simulink model "generic_Truck_And_Trailer"  (R2025a)
settings: Solver=VariableStepAuto  StartTime=0.0  StopTime=350  FixedStep=0.01  MaxStep=0.001  RelTol=1e-3  EnableMultiTasking=on
libraries: TruckMaker4SL x250, simulink x1
(part 6 of 11)

== system generic_Truck_And_Trailer/TruckMaker/IPG Vehicle/CarAndTrailer/Forces/Suspension Forces/Stabi CreateBus CtrlOutOpt ==
  note: <Your model here>
  In : Inport
  Bus Creator{,1..3,11..14,19..22} (12 alike) : BusCreator  Inputs=4
  Bus Creator9 : BusCreator  Inputs=12
  Demux : Demux  Outputs=12
  Demux{2..5,10..13,18..21} (12 alike) : Demux
  Out : Outport
  wires:
  Demux/8 -> Demux13/1  "FR2"
  Demux19/1 -> Bus Creator20/1  "RR3 CtrlOutOpt0"
  Demux19/3 -> Bus Creator20/3  "RR3 CtrlOutOpt2"
  Demux18/4 -> Bus Creator19/4  "RL3 CtrlOutOpt3"
  Demux2/3 -> Bus Creator/3  "FL CtrlOutOpt2"
  Demux4/4 -> Bus Creator2/4  "RL CtrlOutOpt3"
  Demux3/2 -> Bus Creator1/2  "FR CtrlOutOpt1"
  Bus Creator11/1 -> Bus Creator9/5
  Demux2/4 -> Bus Creator/4  "FL CtrlOutOpt3"
  Demux/9 -> Demux18/1  "RL3"
  Demux10/3 -> Bus Creator11/3  "RL2 CtrlOutOpt2"
  Demux2/1 -> Bus Creator/1  "FL CtrlOutOpt0"
  Demux13/4 -> Bus Creator14/4  "FR2 CtrlOutOpt3"
  Demux19/4 -> Bus Creator20/4  "RR3 CtrlOutOpt3"
  Bus Creator1/1 -> Bus Creator9/2
  Bus Creator14/1 -> Bus Creator9/8
  Demux4/3 -> Bus Creator2/3  "RL CtrlOutOpt2"
  Demux2/2 -> Bus Creator/2  "FL CtrlOutOpt1"
  Demux5/1 -> Bus Creator3/1  "RR CtrlOutOpt0"
  Demux18/3 -> Bus Creator19/3  "RL3 CtrlOutOpt2"
  Demux12/1 -> Bus Creator13/1  "FL2 CtrlOutOpt0"
  Demux12/3 -> Bus Creator13/3  "FL2 CtrlOutOpt2"
  Bus Creator19/1 -> Bus Creator9/9
  Demux4/1 -> Bus Creator2/1  "RL CtrlOutOpt0"
  Demux10/1 -> Bus Creator11/1  "RL2 CtrlOutOpt0"
  Bus Creator/1 -> Bus Creator9/1
  Demux11/1 -> Bus Creator12/1  "RR2 CtrlOutOpt0"
  Demux20/1 -> Bus Creator21/1  "RL4 CtrlOutOpt0"
  Demux10/4 -> Bus Creator11/4  "RL2 CtrlOutOpt3"
  Bus Creator12/1 -> Bus Creator9/6
  Demux12/2 -> Bus Creator13/2  "FL2 CtrlOutOpt1"
  Demux11/3 -> Bus Creator12/3  "RR2 CtrlOutOpt2"
  Demux3/4 -> Bus Creator1/4  "FR CtrlOutOpt3"
  Demux18/2 -> Bus Creator19/2  "RL3 CtrlOutOpt1"
  Demux5/3 -> Bus Creator3/3  "RR CtrlOutOpt2"
  Demux19/2 -> Bus Creator20/2  "RR3 CtrlOutOpt1"
  Bus Creator20/1 -> Bus Creator9/10
  Demux20/2 -> Bus Creator21/2  "RL4 CtrlOutOpt1"
  Demux/7 -> Demux12/1  "FL2"
  Bus Creator2/1 -> Bus Creator9/3
  Demux/4 -> Demux5/1  "RR"
  Demux/1 -> Demux2/1  "FL"
  Demux20/4 -> Bus Creator21/4  "RL4 CtrlOutOpt3"
  Demux13/1 -> Bus Creator14/1  "FR2 CtrlOutOpt0"
  Demux/3 -> Demux4/1  "RL"
  Demux20/3 -> Bus Creator21/3  "RL4 CtrlOutOpt2"
  Demux3/1 -> Bus Creator1/1  "FR CtrlOutOpt0"
  Demux21/4 -> Bus Creator22/4  "RR4 CtrlOutOpt3"
  Demux11/4 -> Bus Creator12/4  "RR2 CtrlOutOpt3"
  Demux3/3 -> Bus Creator1/3  "FR CtrlOutOpt2"
  Demux18/1 -> Bus Creator19/1  "RL3 CtrlOutOpt0"
  Demux/10 -> Demux19/1  "RR3"
  Demux10/2 -> Bus Creator11/2  "RL2 CtrlOutOpt1"
  Demux12/4 -> Bus Creator13/4  "FL2 CtrlOutOpt3"
  Demux13/3 -> Bus Creator14/3  "FR2 CtrlOutOpt2"
  Demux4/2 -> Bus Creator2/2  "RL CtrlOutOpt1"
  Demux21/2 -> Bus Creator22/2  "RR4 CtrlOutOpt1"
  Demux5/2 -> Bus Creator3/2  "RR CtrlOutOpt1"
  Bus Creator3/1 -> Bus Creator9/4
  Demux21/3 -> Bus Creator22/3  "RR4 CtrlOutOpt2"
  Demux21/1 -> Bus Creator22/1  "RR4 CtrlOutOpt0"
  Demux/6 -> Demux11/1  "RR2"
  Demux/2 -> Demux3/1  "FR"
  Demux11/2 -> Bus Creator12/2  "RR2 CtrlOutOpt1"
  Demux13/2 -> Bus Creator14/2  "FR2 CtrlOutOpt1"
  Demux/5 -> Demux10/1  "RL2"
  Bus Creator13/1 -> Bus Creator9/7
  Demux5/4 -> Bus Creator3/4  "RR CtrlOutOpt3"
  In/1 -> Demux/1
  Bus Creator9/1 -> Out/1
  Demux/11 -> Demux20/1  "RL4"
  Bus Creator21/1 -> Bus Creator9/11
  Demux/12 -> Demux21/1  "RR4"
  Bus Creator22/1 -> Bus Creator9/12

== matlab function generic_Truck_And_Trailer/TruckMaker/Two_TRack_Model/EKF_ONE_TRACK ==
  data: z input; u input; xhat output; Q input; R input; Ts input; P output; Fyf output; Fyr output
function [xhat, P,Fyf,Fyr] = EKF_Bicycle_Full_NoBias(z, u, Q, R, Ts)
% EKF for One-Track / Bicycle Model (No IMU Bias)
% States: x = [vx; vy; r; Cf; Cr]
% Measurements: z = [ax; ay; vx; vy; r; wL; wR]

%% ---------------- Persistent safe initialization ----------------
persistent x Pk initialized

% Säker initialisering
if isempty(x)
    x = [15; 0; 0.05; 2e4; 2e4];  % vx, vy, r, Cf, Cr
end

if isempty(Pk)
    Pk = diag([1 1 0.05 4e4 4e4].^2); % 5x5
end

if isempty(initialized)
    initialized = true;
end


%% ---------------- Vehicle parameters ----------------


%% ---------------- Inputs ----------------
delta = u(1); % steering angle
Fx    = u(2)/Rw;    % longitudinal force

% PARAMETERS
m  = 6800;        %  mass
g  = 9.82;        % gravity contanst   
Jz = 12994.917;   % yaw interia
Rw = 0.49;          % wheel radius
width = 2.49;       % track width

p_cog  = [3.473; 0; 0.925];
p_fax  = [4.520; 0; 0.490];

p_rax  = [0.950; 0; 0.490];
p_imu  = [3.600; 0; 1.000];

lf = abs(p_fax(1)-p_cog(1));   % front CoG distance
lr = abs(p_cog(1)-p_rax(1));   % rear CoG distance
L  = lf + lr;
h  = p_cog(3);

Rfax = p_fax - p_imu; Rfax(3) = -p_imu(3);
Rrax = p_rax - p_imu; Rrax(3) = -p_imu(3);
Rcog = p_cog - p_imu;


% INPUTS
delta = u(1);                             % Average steering Angle (FL +FR)/2
T_rl  = u(2);                             % torque RL  
T_rr  = u(3);                             %torque RR
Rwheel = 0.49;                            % wheel radius
Fx_vehicle = (T_rl + T_rr)/Rwheel;        % longitudinal force

%% ---------------- States ----------------
vx = x(1); vy = x(2); r = x(3); Cf = x(4); Cr= x(5);

Rotf = [ cos(delta)     -sin(delta)     0;
         sin(delta)      cos(delta)     0;
             0              0           1];

v_cog = [vx; vy; 0];
omega = [0;0;r];

% Contact patch velocities
vf = Rotf.' * (v_cog + cross(omega,Rfax));
vr = v_cog + cross(omega,Rrax);

alpha_f = atan2(vf(2), max(abs(vf(1)),0.1));
alpha_r = atan2(vr(2), max(abs(vr(1)),0.1));

% Longitudinal accel estimate to compute the vertikel forces
dvx_temp = Fx_vehicle/m + vy*r;

% Normal forces
Ffz = m*g*lr/L - m*dvx_temp*h/L;
Frz = m*g*lf/L + m*dvx_temp*h/L;

% Tire forces
Fy_f = Cf * alpha_f * Ffz;
Fy_r = Cr * alpha_r * Frz;

% Full dynamics 
dvx = (Fx_vehicle - Fy_f*sin(delta))/m + vy*r;
dvy = (Fy_f*cos(delta) + Fy_r)/m - vx*r;
dr  = (lf*Fy_f*cos(delta) - lr*Fy_r)/Jz;

% State propagation
xdot = [dvx; dvy; dr; 0; 0];
x_pred = x + Ts*xdot;

%% ---------------- Jacobian F ----------------
F= zeros(5,5);
F(1,:) = [                                1 - (Cf*Ts*sin(delta)*(vy + lf*r))/(m*vx^2),              Ts*(r + (Cf*sin(delta))/(m*vx)),                   Ts*(vy + (Cf*lf*sin(delta))/(m*vx)),    -(Ts*sin(delta)*(delta - (vy + lf*r)/vx))/m,                            0];
F(2,:) = [  -Ts*(r - ((Cr*(vy - lr*r))/vx^2 + (Cf*cos(delta)*(vy + lf*r))/vx^2)/m),      1 - (Ts*(Cr/vx + (Cf*cos(delta))/vx))/m,    -Ts*(vx - ((Cr*lr)/vx - (Cf*lf*cos(delta))/vx)/m),     (Ts*cos(delta)*(delta - (vy + lf*r)/vx))/m,    -(Ts*(vy - lr*r))/(m*vx)];
F(3,:) = [-(Ts*((Cr*lr*(vy - lr*r))/vx^2 - (Cf*lf*cos(delta)*(vy + lf*r))/vx^2))/Jz, (Ts*((Cr*lr)/vx - (Cf*lf*cos(delta))/vx))/Jz, 1 - (Ts*((Cf*cos(delta)*lf^2)/vx + (Cr*lr^2)/vx))/Jz, (Ts*lf*cos(delta)*(delta - (vy + lf*r)/vx))/Jz, (Ts*lr*(vy - lr*r))/(Jz*vx)];
F(4,:) = [                                                                            0,                                              0,                                                      0,                                                 1,                            0];
F(5,:) = [                                                                            0,                                              0,                                                      0,                                                 0,                            1];


%% ---------------- Covariance prediction ----------------
P_pred = F*Pk*F' + Q;

%% ---------------- Measurement model ----------------
ax_hat = dvx -  vy*r;                % longitudinal accel
ay_hat = dvy + vx*r;                % lateral accel
vx_hat = vx;
vy_hat = vy;
r_hat  = r;
wL_hat = (vx - width/2 * r)/Rw;
wR_hat = (vx + width/2 * r)/Rw;

a_cog = [ax_hat; ay_hat; 0];
alpha_vec = [0;0;dr];

% Transform to IMU
a_imu = a_cog - cross(omega, cross(omega,Rcog))- cross(alpha_vec,Rcog);
v_imu = v_cog + cross(omega,Rcog);

z_hat = [a_imu(1:2);
         v_imu(1:2);
         alpha_vec(3);
         omega(3)];

%z_hat = [ax_hat; ay_hat; vx_hat; vy_hat; dr_hat r_hat; wL_hat; wR_hat];

%% ---------------- Measurement Jacobian H ----------------
H = zeros(size(z_hat,1),size(x,1));

%H = zeros(7,5);
H(1,:) = [                               1 - (Cf*Ts*sin(delta)*(vy + lf*r))/(m*vx^2),         Ts*(r + (Cf*sin(delta))/(m*vx)) - r,                      Ts*(vy + (Cf*lf*sin(delta))/(m*vx)) - vy, -(Ts*sin(delta)*(delta - (vy + lf*r)/vx))/m,                            0];
H(2,:) = [-Ts*(r - ((Cr*(vy - lr*r))/vx^2 + (Cf*cos(delta)*(vy + lf*r))/vx^2)/m), 1 - (Ts*(Cr/vx_eff + (Cf*cos(delta))/vx))/m, vx - Ts*(vx - ((Cr*lr)/vx - (Cf*lf*cos(delta))/vx)/m),  (Ts*cos(delta)*(delta - (vy + lf*r)/vx))/m, -(Ts*(vy - lr*r))/(m*vx)];
H(3,:) = [                                                                             1,                                               0,                                                                 0,                                               0,            0];
H(4,:) = [                                                                             0,                                               1,                                                                 0,                                               0,            0];
H(5,:) = [                                                                             0,                                               0,                                                                 0,                                               0,            0];
H(6,:) = [                                                                             0,                                               0,                                                                 1,                                               0,            0];
H(7,:) = [                                                                             1/Rw,                                            0,                                                     -width/(2*Rw),                                               0,            0];
H(8,:) = [                                                                             1/Rw,                                            0,                                                      width/(2*Rw),                                               0,            0];

%% ---------------- EKF update ----------------
S = H*P_pred*H' + R;
K = P_pred*H'/S;

x = x_pred + K*(z - z_hat);
Pk = P_pred - K*S*K';

%% ---------------- Output ----------------
xhat = x;
P = Pk;

end

== matlab function generic_Truck_And_Trailer/TruckMaker/Two_TRack_Model/MATLAB Function2 ==
  data: z input; u input; vx output; Ts input; vy output; wz output; Cf_est output; Cr_est output; Fyf output; Fyr output
function [vx, vy, wz, Cf_est, Cr_est, Fyf, Fyr] = AdaptiveOneTrackCFCR(z, u, Ts)
% Adaptive one-track model for online estimation of front/rear cornering stiffness
%
% Inputs:
%   z  = [ax; ay; vx; vy; wz] -> sensor measurements
%   u  = [delta; Fx]          -> steering angle (rad), longitudinal force (N)
%   Ts -> sampling time (s)
%
% Outputs:
%   vx, vy, wz      -> vehicle states (m/s, m/s, rad/s)
%   Cf_est, Cr_est  -> estimated front/rear cornering stiffness (N/rad)
%   Fyf, Fyr        -> lateral forces (N)

persistent Cf Cr vx_prev vy_prev wz_prev

%% ---------------- Initialization ----------------
if isempty(vx_prev)
    vx_prev = z(3); vy_prev = z(4); wz_prev = z(5);
end
if isempty(Cf)
    Cf = 15000;  % initial guess
    Cr = 15000;
end

%% ---------------- Vehicle parameters ----------------
m  = 7000;      % mass [kg]
Jz = 14232.357; % yaw inertia [kg*m^2]
lf = 1.12;      % front CoG to axle [m]
lr = 2.45;      % rear CoG to axle [m]
Rw = 0.49;      % wheel radius [m]
track = 2.49;   % track width [m]

%% ---------------- Inputs ----------------
delta = u(1); % steering [rad]
Fx    = u(2); % longitudinal force [N]

%% ---------------- States from sensors ----------------
vx = z(3); 
vy = z(4); 
wz = z(5);

% Protect low velocity
vx_eff = max(abs(vx), 1);

%% ---------------- Slip angles ----------------
alpha_f = (vy + lf*wz)/vx_eff - delta;
alpha_r = (vy - lr*wz)/vx_eff;

%% ---------------- Lateral forces ----------------
Fyf = -Cf * alpha_f;
Fyr = -Cr * alpha_r;

%% ---------------- Approximate derivatives ----------------
% simple backward difference
dv_y = (vy - vy_prev)/Ts;
dw_z = (wz - wz_prev)/Ts;

%% ---------------- Regression for Cf/Cr ----------------
% Linear regression: y = Phi * [Cf; Cr]
y   = [m*(dv_y + vx*wz); Jz*dw_z];
Phi = [alpha_f, alpha_r; lf*alpha_f, -lr*alpha_r];

% Adaptive gain
gamma = 1e3;

theta = [Cf; Cr] + gamma * Phi' * (y - Phi*[Cf; Cr]) * Ts;

% Limit to physical range
Cf = theta(1);%max(min(theta(1), 1e5), 5000);
Cr = theta(2);%max(min(theta(2), 1e5), 5000);

Cf_est = Cf;
Cr_est = Cr;

%% ---------------- Recompute lateral forces ----------------
Fyf = Cf_est * alpha_f;
Fyr = -Cr_est * alpha_r;

%% ---------------- Update previous states ----------------
vx_prev = vx;
vy_prev = vy;
wz_prev = wz;

end

== matlab function generic_Truck_And_Trailer/TruckMaker/Comparison Block Forces /Comparison Functions  ==
  data: Vec_v input; alpha_f output; Car_w input; delta_f input; Toe_angle input; alpha_r output; CyF input; CyR input; Fy output; Vx_wheel output; Vy_wheel output
function [alpha_f, alpha_r, Fy, Vx_wheel, Vy_wheel] = tire_model_4W_vehicleFrame(Vec_v, Car_w, delta_f,Toe_angle, CyF, CyR)
%TIRE_MODEL_4W_VEHICLEFRAME
%  Beräknar slipvinklar och lateral forces för ett 4-hjuls fordon
%  
%  Input:
%    Vec_v   - [3x1] Vehicle velocity i vehicle frame [Vx; Vy; Vz]
%    Car_w   - [3x1] Vehicle angular rates i vehicle frame [rollRate; pitchRate; yawRate]
%    delta_f - [2x1] Framhjul styrvinklar [delta_FL; delta_FR] (rad)
%    CyF     - [2x1] Framhjul cornering stiffness per wheel
%    CyR     - [2x1] Bakhjul cornering stiffness per wheel
%
%  Output:
%    alpha_f - [2x1] Slipvinkel framhjul [rad]
%    alpha_r - [2x1] Slipvinkel bakhjul [rad]
%    Fy      - [4x1] Lateral force per wheel [N]
%    Vx_wheel, Vy_wheel - [4x1] Hjulhastigheter i hjulens frame

%% ================= PARAMETERS =================
eps_v  = 0.1;   % min velocity för slipvinkel
g = 9.82;       % gravitation [m/s^2]
load_front_axle = 4805.882;   
load_rear_axle  = 2194.118;   

%% ================= GEOMETRY =================
% Kontaktpunkter i vehicle frame
tire_contact_point_FL = [4.52;  1.05; 0]; 
tire_contact_point_FR = [4.52; -1.05; 0];
tire_contact_point_RL = [0.95;  1.05; 0];
tire_contact_point_RR = [0.95; -1.05; 0];

% Reference point (IMU/vehicle CoM)
Vec_coor = [3.6; 0; 1];

% Vektorer från CoM till hjul
rFL = tire_contact_point_FL - Vec_coor;
rFR = tire_contact_point_FR - Vec_coor;
rRL = tire_contact_point_RL - Vec_coor;
rRR = tire_contact_point_RR - Vec_coor;

%% ================= CONTACT PATCH VELOCITY =================
V_FL = Vec_v + cross(Car_w, rFL);
V_FR = Vec_v + cross(Car_w, rFR);
V_RL = Vec_v + cross(Car_w, rRL);
V_RR = Vec_v + cross(Car_w, rRR);

%% ================= TRANSFORM TO WHEEL FRAME =================
% 2D rotation för framhjul
R_FL = [cos(delta_f(1)), sin(delta_f(1));
       -sin(delta_f(1)), cos(delta_f(1))];

R_FR = [cos(delta_f(2)), sin(delta_f(2));
       -sin(delta_f(2)), cos(delta_f(2))];

% Bakhjul (delta=0)
R_RL = eye(2);
R_RR = eye(2);

% Transformera
V_FL_local = R_FL * V_FL(1:2);
V_FR_local = R_FR * V_FR(1:2);
V_RL_local = R_RL * V_RL(1:2);
V_RR_local = R_RR * V_RR(1:2);


Vx_wheel = [V_FL_local(1); V_FR_local(1); V_RL_local(1); V_RR_local(1)];
Vy_wheel = [V_FL_local(2); V_FR_local(2); V_RL_local(2); V_RR_local(2)];

%% ================= SLIP ANGLES =================
Vx_safe = max(abs(Vx_wheel), eps_v);  % förhindrar division med 0
alpha = atan2(Vy_wheel, Vx_safe);

% Fram och bak separering
alpha_f = alpha(1:2); % - Toe_angle(1:2);
alpha_r = alpha(3:4);% + Toe_angle(3:4).*[1;-1];

%% ================= CORNERING STIFFNESS =================
Cy_FL = CyF(1) * load_front_axle * g / 2;
Cy_FR = CyF(2) * load_front_axle * g / 2;

Cy_RL = CyR(1) * load_rear_axle  * g / 2;
Cy_RR = CyR(2) * load_rear_axle  * g / 2;

Cy = [Cy_FL; Cy_FR; Cy_RL; Cy_RR];

%% ================= LATERAL FORCES =================
Fy = -Cy .* alpha;

end

== matlab function generic_Truck_And_Trailer/TruckMaker/Two_TRack_Model/MATLAB Function3 ==
  data: z input; u input; xhat output; Q input; R input; Ts input; P output; sensor_pos input; F_wheel_pos input; R_wheel_pos input
function [xhat,P] = UKF_5state_4W(z,u,Q,R,Ts,sensor_pos,F_wheel_pos,R_wheel_pos)
% UKF for 4-wheel vehicle
% States: x = [vx; vy; wz; CyF; CyR]
% Measurements: z = [ax; ay; vx; vy; wz; wFL; wFR; wRL; wRR]

persistent x Pk
if isempty(x)
    x = [15; 0; 0.05; 4e4; 4e4]; % initial state
end
if isempty(Pk)
    Pk = diag([1 1 0.01 1e6 1e6]);
end

%% Vehicle parameters
m  = 7000;
Jz = 14232.357;
Rw = 0.49;
g  = 9.82;
track = 2.49;

n = length(x); % state dimension

delta = u(1);      % steering input
Fx_in = u(2)/Rw;   % longitudinal force / wheel radius

%% UKF weights (old style)
W0 = 1 - n/3;
Wi = (1-W0)/(2*n);
gamma = sqrt(n/(1-W0));

%% Sigma points
S = chol(Pk,'lower');
X = zeros(n,2*n+1);
X(:,1) = x;
for i=1:n
    X(:,i+1)   = x + gamma*S(:,i);
    X(:,i+1+n) = x - gamma*S(:,i);
end

%% ------------------- PREDICTION -------------------
X_pred = zeros(n,2*n+1);

for k=1:2*n+1
    vx  = X(1,k);
    vy  = X(2,k);
    wz  = X(3,k);
    CyF = X(4,k);
    CyR = X(5,k);

    Car_v = [vx; vy; 0];
    Car_w = [wx; wy; wz];

    % ---- Wheel velocities at contact patch ----
    V_FL = Car_v + cross(Car_w, F_wheel_pos.FL);
    V_FR = Car_v + cross(Car_w, F_wheel_pos.FR);
    V_RL = Car_v + cross(Car_w, R_wheel_pos.RL);
    V_RR = Car_v + cross(Car_w, R_wheel_pos.RR);

    % ---- Rotate front wheels to wheel frame ----
    R_FL = [ cos(delta)  sin(delta) 0;
            -sin(delta)  cos(delta) 0;
             0           0          1];
    R_FR = R_FL;

    VwfL = R_FL * V_FL;
    VwfR = R_FR * V_FR;

    VwrL = V_RL; % rear wheels no steering
    VwrR = V_RR;

    % ---- Slip angles ----
    alpha_FL = atan2(VwfL(2), VwfL(1));
    alpha_FR = atan2(VwfR(2), VwfR(1));
    alpha_RL = atan2(VwrL(2), VwrL(1));
    alpha_RR = atan2(VwrR(2), VwrR(1));

    % ---- Lateral forces ----
    Fy_FL = -CyF * alpha_FL;
    Fy_FR = -CyF * alpha_FR;
    Fy_RL = -CyR * alpha_RL;
    Fy_RR = -CyR * alpha_RR;

    % Total lateral force & yaw moment
    Fy_total = Fy_FL + Fy_FR + Fy_RL + Fy_RR;
    Mz = F_wheel_pos.FL(1)*Fy_FL + F_wheel_pos.FR(1)*Fy_FR + ...
         R_wheel_pos.RL(1)*Fy_RL + R_wheel_pos.RR(1)*Fy_RR;

    % ---- Dynamics ----
    dvx = Fx_in/m + vy*wz;
    dvy = Fy_total/m - vx*wz;
    dwz = Mz / Jz;

    % Propagate state
    X_pred(:,k) = [vx + Ts*dvx;
                   vy + Ts*dvy;
                   wz + Ts*dwz;
                   CyF;
                   CyR];
end

%% Predicted mean
x_pred = W0*X_pred(:,1);
for k=2:2*n+1
    x_pred = x_pred + Wi*X_pred(:,k);
end

%% Predicted covariance
P_pred = Q;
for k=1:2*n+1
    w = Wi; if k==1, w=W0; end
    dx = X_pred(:,k) - x_pred;
    P_pred = P_pred + w*(dx*dx');
end

%% ------------------- MEASUREMENT -------------------
m_dim = length(z);
Z = zeros(m_dim,2*n+1);

for k=1:2*n+1
    vx  = X_pred(1,k);
    vy  = X_pred(2,k);
    wz  = X_pred(3,k);
    CyF = X_pred(4,k);
    CyR = X_pred(5,k);

    Car_v = [vx; vy; 0];
    Car_w = [0; 0; wz];

    % Velocity at sensor
    V_sensor = Car_v + cross(Car_w, sensor_pos);

    % Acceleration at sensor (approx)
    ax_s = Fx_in/m + vy*wz;
    ay_s = ( -CyF*(atan2(Car_v(2)+wz*F_wheel_pos.FL(2),Car_v(1))) ...
           -CyF*(atan2(Car_v(2)+wz*F_wheel_pos.FR(2),Car_v(1))) ...
           -CyR*(atan2(Car_v(2)+wz*R_wheel_pos.RL(2),Car_v(1))) ...
           -CyR*(atan2(Car_v(2)+wz*R_wheel_pos.RR(2),Car_v(1))) )/m;
    az_s = 0;

    % Wheel speeds
    wFL = V_FL(1)/Rw;
    wFR = V_FR(1)/Rw;
    wRL = V_RL(1)/Rw;
    wRR = V_RR(1)/Rw;

    Z(:,k) = [ax_s; ay_s; vx; vy; wz; wFL; wFR; wRL; wRR];
end

% Predicted measurement mean
z_pred = W0*Z(:,1);
for k=2:2*n+1
    z_pred = z_pred + Wi*Z(:,k);
end

% Measurement covariance & cross-covariance
S_cov = R;
Pxz   = zeros(n,m_dim);
for k=1:2*n+1
    w = Wi; if k==1, w=W0; end
    dz = Z(:,k) - z_pred;
    dx = X_pred(:,k) - x_pred;
    S_cov = S_cov + w*(dz*dz');
    Pxz   = Pxz + w*(dx*dz');
end

% Kalman gain
K = Pxz / (S_cov + 1e-6*eye(m_dim));

% Update
x  = x_pred + K*(z - z_pred);
Pk = P_pred - K*S_cov*K';

xhat = x;
P    = Pk;

end



%%%%%%%%%%%%%%%%%%%%%%%
function [alpha_f, alpha_r, Ffy, Fry, ...
          VfL, VfR, VrL, VrR] = tire_model_4W( ...
          Car_v, Car_w, delta_f, CyF, CyR)

% ------------------------------------------------------------
% INPUTS
% Car_v   = [vx; vy; vz]      (vehicle body frame)
% Car_w   = [0; 0; wz]        (vehicle body frame)
% delta_f = [delta_L; delta_R] (front steering angles)
% CyF     = [Cy_FL; Cy_FR]
% CyR     = [Cy_RL; Cy_RR]
%
% OUTPUTS
% alpha_f = [alpha_FL; alpha_FR]
% alpha_r = [alpha_RL; alpha_RR]
% Ffy     = [Fy_FL; Fy_FR]
% Fry     = [Fy_RL; Fy_RR]
% VwfL etc = velocities in wheel frame
% ------------------------------------------------------------

%% ================= PARAMETERS =================
R = 0.49;                 % wheel radius
g = 9.82;

load_front_axle = 4805.882;
load_rear_axle  = 2194.118;

%% ================= GEOMETRY =================
% Wheel centers in vehicle body frame
tire_coor_Fl = [4.52;  1.05; 0.49];
tire_coor_FR = [4.52; -1.05; 0.49];
tire_coor_Rl = [0.95;  1.05; 0.49];
tire_coor_RR = [0.95; -1.05; 0.49];

Car_coor = [3.6; 0; 1];

% Position vectors CG → wheel center
rFl = tire_coor_Fl - Car_coor;
rFR = tire_coor_FR - Car_coor;
rRl = tire_coor_Rl - Car_coor;
rRR = tire_coor_RR - Car_coor;

% Move to CONTACT PATCH
rFl = rFl + [0;0;-R];
rFR = rFR + [0;0;-R];
rRl = rRl + [0;0;-R];
rRR = rRR + [0;0;-R];

%% ================= VELOCITIES AT CONTACT =================
VfL = Car_v + cross(Car_w, rFl);
VfR = Car_v + cross(Car_w, rFR);
VrL = Car_v + cross(Car_w, rRl);
VrR = Car_v + cross(Car_w, rRR);

%% ================= ROTATE TO WHEEL FRAME =================
% Front left
R_FL = [ cos(delta_f(1))  -sin(delta_f(1)) 0;
        sin(delta_f(1))  cos(delta_f(1)) 0;
         0                0               1];

% Front right
R_FR = [ cos(delta_f(2))  -sin(delta_f(2)) 0;
       sin(delta_f(2))  cos(delta_f(2)) 0;
         0                0               1];

VfL = R_FL * VfL;
VfR = R_FR * VfR;

% Rear wheels (no steering)
%VrL = VrL;
%VrR = VrR;

%% ================= SLIP ANGLES =================
alpha_FL = atan2(VfL(2), VfL(1)); %- delta_f(1);
alpha_FR = atan2(VfR(2), VfR(1));%- delta_f(2);

alpha_RL = atan2(VrL(2), VrL(1));
alpha_RR = atan2(VrR(2), VrR(1));

alpha_f = [alpha_FL; alpha_FR];
alpha_r = [alpha_RL; alpha_RR];

%% ================= CORNERING STIFFNESS =================
Cy_FL = CyF(1) * load_front_axle * g / 2;
Cy_FR = CyF(2) * load_front_axle * g / 2;

Cy_RL = CyR(1) * load_rear_axle * g/2;
Cy_RR = CyR(2) * load_rear_axle * g/2;

%% ================= LATERAL FORCES =================
Fy_FL = -Cy_FL * alpha_FL;
Fy_FR = -Cy_FR * alpha_FR;

Fy_RL = -Cy_RL * alpha_RL;
Fy_RR = -Cy_RR * alpha_RR;

Ffy = [Fy_FL; Fy_FR];
Fry = [Fy_RL; Fy_RR];

end

== matlab function generic_Truck_And_Trailer/TruckMaker/MATLAB Function1 ==
  data: CarVelocity input; CarOmega input; V_FL output; WheelCamberAngle input
function V_FL = fcn(CarVelocity, CarOmega, WheelCamberAngle)

== matlab function generic_Truck_And_Trailer/TruckMaker/Two_TRack_Model/Two Track Model ==
  data: z input; u input; Q input; R input; xhat output; Ts input; P_out output; Fy_mean output; alpha_mean output; V_FL_whl output; V_FR_whl output; V_RL_whl output; V_RR_whl output
function [xhat,P_out,Fy_mean,alpha_mean,...
          V_FL_whl,V_FR_whl,V_RL_whl,V_RR_whl] ...
          = UKF_4Wheel(z,u,Q,R,Ts)

persistent x P

%% ================= INIT =================
if isempty(x)
    x = [15; 0; 0.01; 4; 4; 4; 4];
end

if isempty(P)
    P = diag([1 1 0.01 1e4 1e4 1e4 1e4]);
end

n = length(x);
m = length(z);

%% ================= VEHICLE =================
m_car = 7000;
Jz = 14232.357;
lf = 4.52;
lr = 0.95;
R_w = 0.49;
track=2.10;

%% ================= INPUTS =================
delta_FL = u(1);
delta_FR = u(2);
delta_RL = 0;
delta_RR = 0;

Fx_FL = u(5)/R_w;
Fx_FR = u(6)/R_w;
Fx_RL = u(7)/R_w;
Fx_RR = u(8)/R_w;

%% ================= ROTATION MATRICES =================
R_FL = [cos(delta_FL) sin(delta_FL);
       -sin(delta_FL) cos(delta_FL)];

R_FR = [cos(delta_FR) sin(delta_FR);
       -sin(delta_FR) cos(delta_FR)];

R_RL = eye(2);
R_RR = eye(2);

%% ================= GEOMETRY =================
tire_FL = [lf;  1.05; 0];
tire_FR = [lf; -1.05; 0];
tire_RL = [lr;  1.05; 0];
tire_RR = [lr; -1.05; 0];

CoM = [3.6; 0; 1];  % Ändra koor till COM (Jobba i CoG)  

rFL = tire_FL - CoM;
rFR = tire_FR - CoM;
rRL = tire_RL - CoM;
rRR = tire_RR - CoM;

%% ================= UKF =================
W0 = 1 - n/3;
Wi = (1 - W0)/(2*n);
gamma = sqrt(n/(1-W0));

%P = (P+P')/2 + 1e-9*eye(n); 
S = chol(P,'lower'); %% kolla upp den igen 

X = zeros(n,2*n+1);
X(:,1) = x;

for i=1:n
    X(:,i+1)   = x + gamma*S(:,i);
    X(:,i+1+n) = x - gamma*S(:,i);
end

%% ================= PROPAGATION =================
X_pred = zeros(n,2*n+1);
Fy_sigma = zeros(4,2*n+1);
alpha_sigma = zeros(4,2*n+1);
% R; M; Jz
for k=1:2*n+1

    vx = X(1,k);
    vy = X(2,k);
    r  = X(3,k);

    Cf_FL = X(4,k);
    Cf_FR = X(5,k);
    Cr_RL = X(6,k);
    Cr_RR = X(7,k);

    % ===== FIX 1: korrekt vx_safe =====
    %vx_safe = vx;

    Vc = [vx; vy; 0]; % vehilce Frame 
    omega = [0;0;r];

    V_FL = Vc + cross(omega,rFL);
    V_FR = Vc + cross(omega,rFR);
    V_RL = Vc + cross(omega,rRL);
    V_RR = Vc + cross(omega,rRR);

    V_FL_l = R_FL*V_FL(1:2);
    V_FR_l = R_FR*V_FR(1:2);
    V_RL_l = V_RL(1:2);
    V_RR_l = V_RR(1:2);
    
    %============Side Slip Vinkel på respektiv däck ==================
    alpha_FL = atan2(V_FL_l(2),max(abs(V_FL_l(1)),0.1));
    alpha_FR = atan2(V_FR_l(2),max(abs(V_FR_l(1)),0.1));
    alpha_RL = atan2(V_RL_l(2),max(abs(V_RL_l(1)),0.1));
    alpha_RR = atan2(V_RR_l(2),max(abs(V_RR_l(1)),0.1));


    %===================Forces==============================
    Fy_FL = -Cf_FL*alpha_FL;
    Fy_FR = -Cf_FR*alpha_FR;
    Fy_RL = -Cr_RL*alpha_RL;
    Fy_RR = -Cr_RR*alpha_RR;


    % Transformerta dessa krafter till kroppens FRAME
    F_FL = R_FL'*[Fx_FL;Fy_FL];
    F_FR = R_FR'*[Fx_FR;Fy_FR];
    F_RL = [Fx_RL;Fy_RL];
    F_RR = [Fx_RR;Fy_RR];

    Fx_sum = F_FL(1)+F_FR(1)+F_RL(1)+F_RR(1);
    Fy_sum = F_FL(2)+F_FR(2)+F_RL(2)+F_RR(2);

    dvx = Fx_sum/m_car + vy*r; % andra terma roteradnde koordinat system 
    dvy = Fy_sum/m_car - vx*r; 

%dW = truck.Jinv * (cross(R1, RotW1*F1) + cross(R2, RotW2*F2) 
                    % + cross(R3, F3) + cross(R4, F4));

    % ===== FIX 2: korrekt  eller ej fråga Axel  yaw moment =====
    % !!!!!!!!!!
    Mz = (lf-CoM(1))*(F_FL(2)+F_FR(2)) - (CoM(1)-lr)*(F_RL(2)+F_RR(2)) ... 
        + (track/2)*(F_FR(1)-F_FL(1)) + (track/2)*(F_RR(1)-F_RL(1));
    dr = Mz / Jz;

    X_pred(:,k) = [vx+dvx*Ts;
                   vy+dvy*Ts;
                   r+dr*Ts;
                   Cf_FL;
                   Cf_FR;
                   Cr_RL;
                   Cr_RR];

    Fy_sigma(:,k)    = [F_FL(2);F_FR(2);F_RL(2);F_RR(2)];
    alpha_sigma(:,k) = [alpha_FL;alpha_FR;alpha_RL;alpha_RR];
end

W = [W0 repmat(Wi,1,2*n)];
%x_pred = X_pred*W';
Fy_mean = Fy_sigma*W';
alpha_mean = alpha_sigma*W';
%% Predicted mean
x_pred = W0*X_pred(:,1);
for k=2:2*n+1
    x_pred = x_pred + Wi*X_pred(:,k);
end

%% ================= COVARIANCE =================
% P_pred = Q*Ts;
% for k=1:2*n+1
%     dx = X_pred(:,k)-x_pred;
%     P_pred = P_pred + W(k)*(dx*dx');
% end

%% Predicted covariance
P_pred = Q*Ts;
for k=1:2*n+1
    w = (k==1)*W0 + (k>1)*Wi;
    dx = X_pred(:,k) - x_pred;
    P_pred = P_pred + w*(dx*dx');
end
%% ================= MEASUREMENT =================
Z_sigma = zeros(m,2*n+1);

for k=1:2*n+1

    vx = X_pred(1,k);
    vy = X_pred(2,k);
    r  = X_pred(3,k);

    %Cf_FL = X_pred(4,k);
    %Cf_FR = X_pred(5,k);
    %Cr_RL = X_pred(6,k);
    %Cr_RR = X_pred(7,k);


    vx_safe = abs(vx);

    Vc = [vx_safe;vy;0];
    omega = [0;0;r];

    V_FL = Vc + cross(omega,rFL);
    V_FR = Vc + cross(omega,rFR);
    V_RL = Vc + cross(omega,rRL);
    V_RR = Vc + cross(omega,rRR);

    V_FL_l = R_FL*V_FL(1:2);
    V_FR_l = R_FR*V_FR(1:2);
    V_RL_l = V_RL(1:2);
    V_RR_l = V_RR(1:2);

     %============Side Slip Vinkel på respektiv däck ==================
    alpha_FL = atan2(V_FL_l(2),max(abs(V_FL_l(1)),0.1));
    alpha_FR = atan2(V_FR_l(2),max(abs(V_FR_l(1)),0.1));
    alpha_RL = atan2(V_RL_l(2),max(abs(V_RL_l(1)),0.1));
    alpha_RR = atan2(V_RR_l(2),max(abs(V_RR_l(1)),0.1));


    %===================Forces==============================
    Fy_FL = -Cf_FL*alpha_FL;
    Fy_FR = -Cf_FR*alpha_FR;
    Fy_RL = -Cr_RL*alpha_RL;
    Fy_RR = -Cr_RR*alpha_RR;


    % Transformerta dessa krafter till kroppens FRAME
    F_FL = R_FL'*[Fx_FL;Fy_FL];
    F_FR = R_FR'*[Fx_FR;Fy_FR];
    F_RL = [Fx_RL;Fy_RL];
    F_RR = [Fx_RR;Fy_RR];

    Fx_sum = F_FL(1)+F_FR(1)+F_RL(1)+F_RR(1);
    Fy_sum = F_FL(2)+F_FR(2)+F_RL(2)+F_RR(2);

    % ===== FIX 3: hjulhastigheter istället för krafter =====
    w_FL = V_FL_l(1)/R_w;    % Fråga MATS om Long slip och R_w 
    w_FR = V_FR_l(1)/R_w;
    w_RL = V_RL_l(1)/R_w;
    w_RR = V_RR_l(1)/R_w;

    ax = (Fx_sum)/m_car ;
    ay = (Fy_sum)/m_car;

    Z_sigma(:,k) = [ax; ay; vx; vy; r; w_FL; w_FR; w_RL; w_RR];
end

% z_pred = Z_sigma*W';
% 
% P_zz = R;
% P_xz = zeros(n,m);
% 
% for k=1:2*n+1
%     dz = Z_sigma(:,k)-z_pred;
%     dx = X_pred(:,k)-x_pred;
%     P_zz = P_zz + W(k)*(dz*dz');
%     P_xz = P_xz + W(k)*(dx*dz');
% end
% 
% %% ================= UPDATE =================
% K =   P_xz / P_zz;
% x = x_pred + K*(z - z_pred);
% 
% P = P_pred - K*P_zz*K';

% ===== FIX 4: symmetrisera P =====
%P = (P+P')/2 + 1e-9*eye(n);

%% Measurement mean
z_pred = W0*Z_sigma(:,1);
for k=2:2*n+1
    z_pred = z_pred + Wi*Z_sigma(:,k);
end

%% Measurement covariance
S_cov = R;
for k=1:2*n+1
    w = (k==1)*W0 + (k>1)*Wi;
    dz = Z_sigma(:,k) - z_pred;
    S_cov = S_cov + w*(dz*dz');
end

%% Cross covariance
Pxz = zeros(n,length(z));
for k=1:2*n+1
    w = (k==1)*W0 + (k>1)*Wi;
    dx = X_pred(:,k) - x_pred;
    dz = Z_sigma(:,k) - z_pred;
    Pxz = Pxz + w*(dx*dz');
end

%% Kalman update
K = Pxz / (S_cov);
x = x_pred + K*(z - z_pred);
P = P_pred - K*S_cov*K';

%% ================= OUTPUT =================
vx = x(1); vy = x(2); r = x(3);

Vc = [vx;vy;0];
omega = [0;0;r];

V_FL = Vc + cross(omega,rFL);
V_FR = Vc + cross(omega,rFR);
V_RL = Vc + cross(omega,rRL);
V_RR = Vc + cross(omega,rRR);

V_FL_whl = R_FL*V_FL(1:2);
V_FR_whl = R_FR*V_FR(1:2);
V_RL_whl = V_RL(1:2);
V_RR_whl = V_RR(1:2);

xhat =  x;
P_out = P;

end

== matlab function generic_Truck_And_Trailer/TruckMaker/Two_TRack_Model/Two Track Model1 ==
  data: z input; u input; Q input; R input; xhat output; Ts input; P_out output; Fy_mean output; alpha_mean output; V_FL_whl output; V_FR_whl output; V_RL_whl output; V_RR_whl output
function [xhat,P_out,Fy_mean,alpha_mean,...
          V_FL_whl,V_FR_whl,V_RL_whl,V_RR_whl] ...
          = UKF_4Wheel(z,u,Q,R,Ts)

persistent x P

%% ================= INIT =================
if isempty(x)
    x = [15; 0; 0.01; 10; 10; 10; 10];  % startvärden på cornering stiffness
end

if isempty(P)
    P = diag([1 1 0.01 1 1 1 1]);
end

n = length(x);
m = length(z);

%% ================= VEHICLE =================
m_car = 7000;
Jz = 14232.357;
lf = 4.52;
lr = 0.95;
R_w = 0.49;
track=2.10;
h_CoM = 1;  % höjd på CoM

%% ================= INPUTS =================
delta_FL = u(1);
delta_FR = u(2);
delta_RL = 0;
delta_RR = 0;

Fx_FL = u(5)/R_w;
Fx_FR = u(6)/R_w;
Fx_RL = u(7)/R_w;
Fx_RR = u(8)/R_w;

%% ================= ROTATION MATRICES =================
R_FL = [cos(delta_FL) sin(delta_FL);
       -sin(delta_FL) cos(delta_FL)];

R_FR = [cos(delta_FR) sin(delta_FR);
       -sin(delta_FR) cos(delta_FR)];

R_RL = eye(2);
R_RR = eye(2);

%% ================= GEOMETRY =================
tire_FL = [lf;  track/2; 0];
tire_FR = [lf; -track/2; 0];
tire_RL = [lr;  track/2; 0];
tire_RR = [lr; -track/2; 0];

CoM = [3.6; 0; h_CoM];  

rFL = tire_FL - CoM;
rFR = tire_FR - CoM;
rRL = tire_RL - CoM;
rRR = tire_RR - CoM;

%% ================= UKF =================
W0 = 1 - n/3;
Wi = (1 - W0)/(2*n);
gamma = sqrt(n/(1-W0));

S = chol(P,'lower');

X = zeros(n,2*n+1);
X(:,1) = x;

for i=1:n
    X(:,i+1)   = x + gamma*S(:,i);
    X(:,i+1+n) = x - gamma*S(:,i);
end

%% ================= PROPAGATION =================
X_pred = zeros(n,2*n+1);
Fy_sigma = zeros(4,2*n+1);
alpha_sigma = zeros(4,2*n+1);

for k=1:2*n+1

    vx = X(1,k);
    vy = X(2,k);
    r  = X(3,k);

    Cf_FL = X(4,k);
    Cf_FR = X(5,k);
    Cr_RL = X(6,k);
    Cr_RR = X(7,k);

    Vc = [vx; vy; 0];
    omega = [0;0;r];

    V_FL = Vc + cross(omega,rFL);
    V_FR = Vc + cross(omega,rFR);
    V_RL = Vc + cross(omega,rRL);
    V_RR = Vc + cross(omega,rRR);

    V_FL_l = R_FL*V_FL(1:2);
    V_FR_l = R_FR*V_FR(1:2);
    V_RL_l = V_RL(1:2);
    V_RR_l = V_RR(1:2);
    
    % Side slip angles
    alpha_FL = atan2(V_FL_l(2),max(abs(V_FL_l(1)),0.1));
    alpha_FR = atan2(V_FR_l(2),max(abs(V_FR_l(1)),0.1));
    alpha_RL = atan2(V_RL_l(2),max(abs(V_RL_l(1)),0.1));
    alpha_RR = atan2(V_RR_l(2),max(abs(V_RR_l(1)),0.1));

    % ================= LOAD TRANSFER =================
    Fz_FL = m_car/4*9.81 - m_car*r*vy - m_car*vx^2*lr/(lf+lr); % enkel approx
    Fz_FR = m_car/4*9.81 - m_car*r*vy - m_car*vx^2*lr/(lf+lr);
    Fz_RL = m_car/4*9.81 + m_car*r*vy + m_car*vx^2*lf/(lf+lr);
    Fz_RR = m_car/4*9.81 + m_car*r*vy + m_car*vx^2*lf/(lf+lr);

    % ================= FORCES =================
    Fy_FL = -Cf_FL * Fz_FL * alpha_FL;
    Fy_FR = -Cf_FR * Fz_FR * alpha_FR;
    Fy_RL = -Cr_RL * Fz_RL * alpha_RL;
    Fy_RR = -Cr_RR * Fz_RR * alpha_RR;

    F_FL = R_FL'*[Fx_FL;Fy_FL];
    F_FR = R_FR'*[Fx_FR;Fy_FR];
    F_RL = [Fx_RL;Fy_RL];
    F_RR = [Fx_RR;Fy_RR];

    Fx_sum = F_FL(1)+F_FR(1)+F_RL(1)+F_RR(1);
    Fy_sum = F_FL(2)+F_FR(2)+F_RL(2)+F_RR(2);

    dvx = Fx_sum/m_car + vy*r;
    dvy = Fy_sum/m_car - vx*r;

    Mz = (lf-CoM(1))*(F_FL(2)+F_FR(2)) - (CoM(1)-lr)*(F_RL(2)+F_RR(2)) ...
        + (track/2)*(F_FR(1)-F_FL(1)) + (track/2)*(F_RR(1)-F_RL(1));
    dr = Mz / Jz;

    X_pred(:,k) = [vx+dvx*Ts;
                   vy+dvy*Ts;
                   r+dr*Ts;
                   Cf_FL;
                   Cf_FR;
                   Cr_RL;
                   Cr_RR];

    Fy_sigma(:,k)    = [F_FL(2);F_FR(2);F_RL(2);F_RR(2)];
    alpha_sigma(:,k) = [alpha_FL;alpha_FR;alpha_RL;alpha_RR];
end

%% ================= UKF MEAN & COVARIANCE =================
W = [W0 repmat(Wi,1,2*n)];
Fy_mean = Fy_sigma*W';
alpha_mean = alpha_sigma*W';

% State mean
x_pred = W0*X_pred(:,1);
for k=2:2*n+1
    x_pred = x_pred + Wi*X_pred(:,k);
end

% State covariance
P_pred = Q*Ts;
for k=1:2*n+1
    w = (k==1)*W0 + (k>1)*Wi;
    dx = X_pred(:,k) - x_pred;
    P_pred = P_pred + w*(dx*dx');
end

%% ================= MEASUREMENT =================
Z_sigma = zeros(m,2*n+1);

for k=1:2*n+1
    vx = X_pred(1,k);
    vy = X_pred(2,k);
    r  = X_pred(3,k);

    Cf_FL = X_pred(4,k);
    Cf_FR = X_pred(5,k);
    Cr_RL = X_pred(6,k);
    Cr_RR = X_pred(7,k);

    Vc = [vx;vy;0];
    omega = [0;0;r];

    V_FL = Vc + cross(omega,rFL);
    V_FR = Vc + cross(omega,rFR);
    V_RL = Vc + cross(omega,rRL);
    V_RR = Vc + cross(omega,rRR);

    V_FL_l = R_FL*V_FL(1:2);
    V_FR_l = R_FR*V_FR(1:2);
    V_RL_l = V_RL(1:2);
    V_RR_l = V_RR(1:2);

    alpha_FL = atan2(V_FL_l(2),max(abs(V_FL_l(1)),0.1));
    alpha_FR = atan2(V_FR_l(2),max(abs(V_FR_l(1)),0.1));
    alpha_RL = atan2(V_RL_l(2),max(abs(V_RL_l(1)),0.1));
    alpha_RR = atan2(V_RR_l(2),max(abs(V_RR_l(1)),0.1));

     % ================= LOAD TRANSFER =================
    Fz_FL = m_car/4*9.81 - m_car*r*vy - m_car*vx^2*lr/(lf+lr); % enkel approx
    Fz_FR = m_car/4*9.81 - m_car*r*vy - m_car*vx^2*lr/(lf+lr);
    Fz_RL = m_car/4*9.81 + m_car*r*vy + m_car*vx^2*lf/(lf+lr);
    Fz_RR = m_car/4*9.81 + m_car*r*vy + m_car*vx^2*lf/(lf+lr);

    Fy_FL = -Cf_FL * Fz_FL * alpha_FL;
    Fy_FR = -Cf_FR * Fz_FR * alpha_FR;
    Fy_RL = -Cr_RL * Fz_RL * alpha_RL;
    Fy_RR = -Cr_RR * Fz_RR * alpha_RR;

    F_FL = R_FL'*[Fx_FL;Fy_FL];
    F_FR = R_FR'*[Fx_FR;Fy_FR];
    F_RL = [Fx_RL;Fy_RL];
    F_RR = [Fx_RR;Fy_RR];

    Fx_sum = F_FL(1)+F_FR(1)+F_RL(1)+F_RR(1);
    Fy_sum = F_FL(2)+F_FR(2)+F_RL(2)+F_RR(2);

    w_FL = V_FL_l(1)/R_w;
    w_FR = V_FR_l(1)/R_w;
    w_RL = V_RL_l(1)/R_w;
    w_RR = V_RR_l(1)/R_w;

    ax = Fx_sum/m_car;
    ay = Fy_sum/m_car;

    Z_sigma(:,k) = [ax; ay; vx; vy; r; w_FL; w_FR; w_RL; w_RR];
end

%% ================= UKF UPDATE =================
% Measurement mean
z_pred = W0*Z_sigma(:,1);
for k=2:2*n+1
    z_pred = z_pred + Wi*Z_sigma(:,k);
end

% Measurement covariance
S_cov = R;
for k=1:2*n+1
    w = (k==1)*W0 + (k>1)*Wi;
    dz = Z_sigma(:,k) - z_pred;
    S_cov = S_cov + w*(dz*dz');
end

% Cross covariance
Pxz = zeros(n,length(z));
for k=1:2*n+1
    w = (k==1)*W0 + (k>1)*Wi;
    dx = X_pred(:,k) - x_pred;
    dz = Z_sigma(:,k) - z_pred;
    Pxz = Pxz + w*(dx*dz');
end

% Kalman update
K = Pxz / S_cov;
x = x_pred + K*(z - z_pred);
P = P_pred - K*S_cov*K';

%% ================= OUTPUT =================
vx = x(1); vy = x(2); r = x(3);

Vc = [vx;vy;0];
omega = [0;0;r];

V_FL = Vc + cross(omega,rFL);
V_FR = Vc + cross(omega,rFR);
V_RL = Vc + cross(omega,rRL);
V_RR = Vc + cross(omega,rRR);

V_FL_whl = R_FL*V_FL(1:2);
V_FR_whl = R_FR*V_FR(1:2);
V_RL_whl = V_RL(1:2);
V_RR_whl = V_RR(1:2);

xhat =  x;
P_out = P;
Fy_mean = Fy_mean;
alpha_mean = alpha_mean;

end

== matlab function generic_Truck_And_Trailer/TruckMaker/Subsystem1/ONE_TRACK_MODEL_TRACTOR_UKF/MATLAB Function ==
  data: z input; u input; Cf output; Cr output; alpha_f output; alpha_r output
function [Cf, Cr, alpha_f, alpha_r] = stiffness_computation(z, u)
%
% Signal: z = [ ax; ay; az; 
%               vx; vy; vz;
%               rx; ry; rz;
%               alphax; alphay; alphaz;
%               wFL; wFR; wRL; wRR; ]
%
%         u = [ delta; T_rl; T_rr; ]
%

% ------------------------------------------------------------------------%
% Physics
% ------------------------------------------------------------------------%

g = 9.82; % [m/s^2]

% ------------------------------------------------------------------------%
% Truck Parameters
% ------------------------------------------------------------------------%

% Mass [kg]
m = 6800;

% Inertial tensor [kg m^2]
J = [
     5430.025, 0.000,    -589.488;
     0.000,    9407.562,  0.000;
    -589.488,  0.000,     12994.917;
];

% Position vectors [m]
p_cog  = [3.473, 0.000, 0.925].';  % Center of Gravity
p_fax  = [4.520, 0.000, 0.490].';  % Front axle
p_rax  = [0.950, 0.000, 0.490].';  % Rear axle
p_bod  = [3.600, 0.000, 1.000].';  % Body frame
p_imu  = p_bod;

% p_wfl  = [4.520,  1.050, 0.490].'; % Front wheel left
% p_wfr  = [4.520, -1.050, 0.490].'; % Front wheel right
% 
% p_wrl  = [0.950,  1.050, 0.490].'; % Rear wheel left
% p_wrcl = [0.950,  0.860, 0.490].'; % Rear wheel carrier left
% p_wrcr = [0.950, -0.860, 0.490].'; % Rear wheel carrier right
% p_wrr  = [0.950, -1.050, 0.490].'; % Rear wheel right
% 
% Axle load
% m_f = 4805.882; % [kg]
% m_r = 2194.118; % [kg]
% 
% Wheel base
% long = [1,0,0] * abs(p_fax - p_rax); % length [m]
% wide = [0,1,0] * abs(p_wrr - p_wrl); % width  [m]

% CoG hight
high = p_cog(3);

% Wheel radius
% Rwf = 0.505;
% Rwr = 0.505;

% longitudinal distance from cog to axles
lf = [1,0,0] * abs(p_fax - p_cog);
lr = [1,0,0] * abs(p_rax - p_cog);

% ------------------------------------------------------------------------%
% Inputs
% ------------------------------------------------------------------------%

a =  [z(1:2);0]; % IMU acceleration
v =  [z(3:4);0]; % IMU velocity

alpha = [0;0;0];     % IMU yaw acceleration

omega = [0;0;z(end)];  % IMU yaw rate


delta = u(1); % steering angle of one-track front wheel (pre-computed)

T_rl = u(2); % rear left  torque (not used)
T_rr = u(3); % rear right torque (not used)
 
% ------------------------------------------------------------------------%
% Translate measurements
% ------------------------------------------------------------------------%

% displacement vectors
Rfax = p_fax - p_imu; Rfax(3) = -p_imu(3); % straight projection to contact
Rrax = p_rax - p_imu; Rrax(3) = -p_imu(3); % --||--
Rcog = p_cog - p_imu;

% rotation matrix
Rotf = [ 
   cos(delta), -sin(delta), 0;
   sin(delta),  cos(delta), 0;
            0,           0, 1;
];

% velocity translation
% --------------------
vf = Rotf.' * (v + cross(omega, Rfax));
vr = eye(3) * (v + cross(omega, Rrax));

% acceleration translation 
% ------------------------
acog = a + cross(omega, cross(omega, Rcog)) + cross(alpha, Rcog);

% ------------------------------------------------------------------------%
% Computation
% ------------------------------------------------------------------------%

% lateral forces
% --------------
%Ffy = (J(3,3)*alpha(3)+m*acog(2)*lr) / (long * cos(delta));
%Fry = (m*acog(2)*lf - J(3,3)*alpha(3)) / long;

Ffy = (acog(2)*lr) / cos(delta);
Fry = (acog(2)*lf);

% slip
% ----
alpha_f = atan2(vf(2), max(abs(vf(1)), .1));
alpha_r = atan2(vr(2), max(abs(vr(1)), .1));

% normal forces
% -------------
%Ffz = m*g*lr/long - m*acog(1)*high/long;
%Frz = m*g*lf/long + m*acog(1)*high/long;

Ffz = g*lr - acog(1)*high;
Frz = g*lf + acog(1)*high;

% normalized coefficients
% -----------------------
Cf = Ffy / (alpha_f * Ffz); % reference 
Cr = Fry / (alpha_r * Frz); % reference
